simulink model "pid3"  (R2020b)
settings: Solver=VariableStepAuto  StartTime=0.0  StopTime=10.0  RelTol=1e-3
undefined symbols (not defined in the file): Kd, Ki, Kp
settings Model: Creator=stkaravind  LastModifiedBy=stkaravind

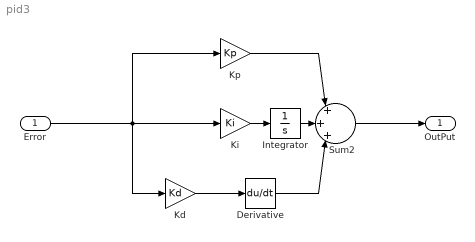
== system pid3 ==
  Error : Inport  OutDataTypeStr=double  PortDimensions=1  SampleTime=0
  Derivative : Derivative
  Integrator : Integrator
  Kd : Gain  Gain=Kd
  Ki : Gain  Gain=Ki
  Kp : Gain  Gain=Kp
  Sum2 : Sum  Inputs=|+|+|+|
  OutPut : Outport  OutDataTypeStr=double  PortDimensions=1  SampleTime=0
  wires:
  Derivative/1 -> Sum2/3
  Error/1 -> Ki/1, Kp/1, Kd/1
  Sum2/1 -> OutPut/1
  Kp/1 -> Sum2/1
  Ki/1 -> Integrator/1
  Integrator/1 -> Sum2/2
  Kd/1 -> Derivative/1
